simulink model "nl_obsv_hydrotrans_dspace"  (R2021b)
settings: Solver=ode1be  StartTime=0.0  StopTime=inf  FixedStep=ts  MaxStep=ts
PostLoadFcn:
  | if any(exist('dsrtsu_mdlpostloadfcn', 'file') ~= 0), dsrtsu_mdlpostloadfcn('Execute', bdroot); end
InitFcn:
  | , if any(exist('rtifpga_mdlclblib', 'file') ~= 0), rtifpga_mdlclblib('Init', bdroot); end,
  | , if any(exist('dsmpb_private', 'file') ~= 0), dsmpb_private('dsmpb_mdlclblib', 'Init', bdroot); end,
values from neighbouring files (symbols this model uses):
  bd = 5e-2    (= 0.05)    [init_nlobsv_hd.m]
  bf = 0.1    [init_nlobsv_hd.m]
  bm = 0.02    [init_nlobsv_hd.m]
  bp = 0.02    [init_nlobsv_hd.m]
  bulk = 8.36e9    (= 8360000000)    [init_nlobsv_hd.m]
  engine_speed_ref_rpm = 1940    [init_nlobsv_hd.m]
  Jm = 0.05    [init_nlobsv_hd.m]
  Jp = 0.05    [init_nlobsv_hd.m]
  kdrag = 0.01    [init_nlobsv_hd.m]
  kdrag_model = 0.01    [init_nlobsv_hd.m]
  ki_engine = 2.5e-1    (= 0.25)    [init_nlobsv_hd.m]
  kleak = 1e-6    (= 1e-06)    [init_nlobsv_hd.m]
  kp_engine = 2.5e-2    (= 0.025)    [init_nlobsv_hd.m]
  max_domega_m_dt = omega_m_nom_rpm/4    (= 1000)    [init_nlobsv_hd.m]
  ntg = 1    [init_nlobsv_hd.m]
  omega_m_nom_rpm = 4000    [init_nlobsv_hd.m]
  omega_m_ref = 3200    [init_nlobsv_hd.m]
  P0 = eye(4)    [init_nlobsv_hd.m]
  q11 = 10    [init_nlobsv_hd.m]
  q22 = 10    [init_nlobsv_hd.m]
  q33 = 10    [init_nlobsv_hd.m]
  q44 = 2e3    (= 2000)    [init_nlobsv_hd.m]
  ts = 1e-3    (= 0.001)    [init_nlobsv_hd.m]
  tstep = 20    [init_nlobsv_hd.m]
  Vm_nom = 280    [init_nlobsv_hd.m]
  Vp_nom = 210    [init_nlobsv_hd.m]
undefined symbols (not defined in the file or in its folder): consumption, DiscIntNeverNeededParam, rpm_base, rpm_consumption, torque_base, torque_consumption, torque_friction_base
libraries: fl_lib x70, nesl_utility x36, linear_swashplate_ctrl_lib x4, variable_displacement_motor_2_lib x2, variable_displacement_pump_2_lib x2, fixed_displacement_pump_lib x2, relief_valve_lib x2, inverse_shuttle_valve_lib x2, engine_speed_ctrl_kinputs_lib x1, ice_lib x1, gear2_lib x1, flexshaft_lib x1
(part 1 of 2)
PreSaveFcn:
  | , if any(exist('dsmpb_private', 'file') ~= 0), dsmpb_private('dsmpb_mdlclblib', 'PreSave', bdroot); end,
CloseFcn:
  | , if any(exist('dsmpb_private', 'file') ~= 0), dsmpb_private('dsmpb_mdlclblib', 'Close', bdroot); end,
settings Model: RTICANMMDATA=struct('GeneralSetupData',struct('modelroot','C:\Users\dbagn\Dropbox\anno_2022_2023\matlab\anno2022\lectures\nonlinear_obsv_hydrostatic_transmission\2022_08_10','generalsettings',struct('filesettings',struct('destfolder',struct('Name','RTICANMM_FILES','Check',1),'buildfolder',struct('Name','.','Check',1),'AbsDestfolder',struct('Name','C:\Users\dbagn\Dropbox\anno_2022_2023\matlab\anno2022\lectures\nonlinear_obsv_hydrostatic_transmission\2022_08_10\RTICANMM_FILES'),'AbsBuildfolder',struct('Name','C:\Users\dbagn\Dropbox\anno_2022_2023\matlab\anno2022\lectures\nonlinear_obsv_hydrostatic_transmission\2022_08_10'))),'options',struct('addpaths',1,'rmpaths',1,'addtrcexclusion',true,'cannavigator',struct('checkmonitoring',0),'show_usrtrc',0,'use_usrtrc',0),'advanced',struct('options',ones(1,100)),'MPSetup',{{}},'RTI',struct('Type','DSRT','Ver','4.6','Date','02-Nov-2021'),'modelname','nl_obsv_hydrotrans_dspace','block','nl_obsv_hydrotrans_dspace'))  DSRTSU_INTERNAL_RTIFPGA=170  DSRTSU_INTERNAL_RTISTBM_VER=1.4.3  DSMPB_ID_DATA={}  SimulationMode=accelerator  Creator=dbagn  LastModifiedBy=dbagn
settings SolverCC: ZeroCrossAlgorithm=Adaptive
settings DataIOCC: SaveOutput=off  SignalLogging=off  DSMLogging=off  SaveTime=off  ReturnWorkspaceOutputs=off
settings OptimizationCC: BlockReduction=off  ConditionallyExecuteInputs=off  OptimizeBlockIOStorage=off  BufferReuse=off  EnhancedBackFolding=on  PassReuseOutputArgsThreshold=0  OptimizeBlockOrder=speed  DifferentSizesBufferReuse=on
settings DebuggingCC: IgnoredZcDiagnostic=none  TasksWithSamePriorityMsg=none  ParameterTunabilityLossMsg=error
settings HardwareCC: ProdBitPerPointer=32  ProdBitPerSizeT=32  ProdBitPerPtrDiffT=32  ProdLargestAtomicInteger=Integer  ProdWordSize=32  ProdLongLongMode=on  ProdHWDeviceType=Custom Processor->Custom
settings ModelReferenceCC: EnableParallelModelReferenceBuilds=on
settings SFSimCC: MATLABDynamicMemAlloc=off
settings RTWCC: Description=dSPACE Run-Time Target (for VEOS on Windows and ConfigurationDesk)  SystemTargetFile=dsrt.tlc  GenCodeOnly=on  MakeCommand=make_dsrt  TemplateMakefile=dsrt_default_tmf  RTWVerbose=off
settings CodeAppCC: ForceParamTrailComments=on  OperatorAnnotations=on
settings STFCustomTargetCC: TargetLangStandard=C99 (ISO)  ParMdlRefBuildCompliant=on  GRTInterface=off  SystemTargetFile=dsrt.tlc
settings GRTTargetCC: CompOptLevelCompliant=off  ConcurrentExecutionCompliant=off  CombineOutputUpdateFcns=off  MatFileLogging=off  CPPClassGenCompliant=off  UseToolchainInfoCompliant=off

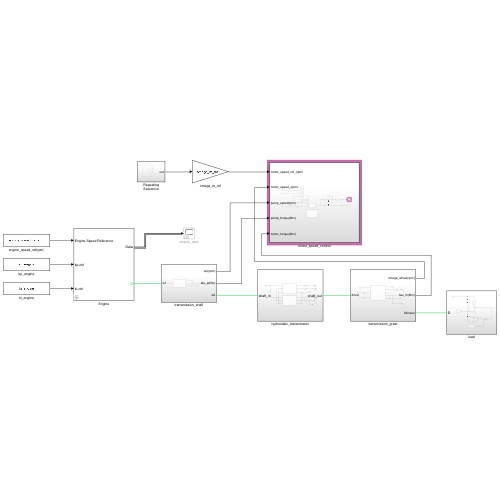
[thumbnail: Simulink's stored preview of the top-level diagram]
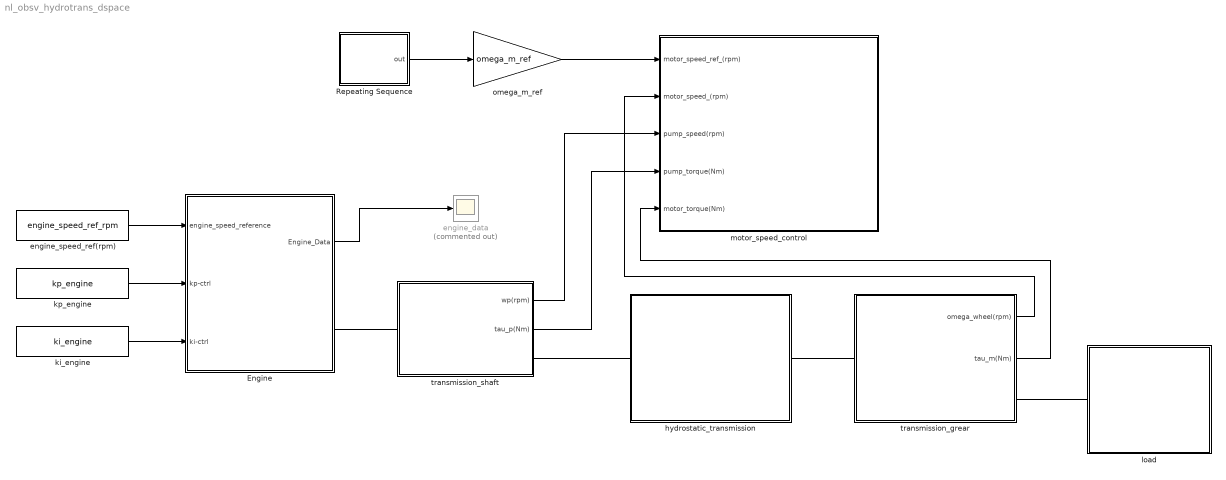
== system nl_obsv_hydrotrans_dspace ==
  Engine : Subsystem  mask(Internal Combustion Engine (ICE)){inertia=7.5, inertia_unit=kg*m^2, init_speed=5, diesel_density=0.85, diesel_density_unit=kg/l, rpm_base=rpm_base, rpm_base_unit=rpm, torque_friction_base=torque_friction_base, torque_friction_base_unit=N*m, torque_base=torque_base, torque_base_unit=N*m, rpm_consumption=rpm_consumption, rpm_consumption_unit=rpm, torque_consumption=torque_consumption, torque_consumption_unit=N*m, consumption=consumption, consumption_unit=g/(kW*hr), kd=0}
      mask prompts: init_speed "Initial Speed (RPM)"; diesel_density "Diesel density"; rpm_base "Base Speed Breakpoints"; torque_friction_base "Base Torque Friction Breakpoints"; torque_base "Base Torque Breakpoints"; rpm_consumption "Speed consumption breakpoints"; torque_consumption "Torque consumption breakpoints"; consumption "Consumption map"
      mask help:
      | This component models a generic internal combustion engine, modelled by means of introducing its characteristic performance maps.
      | Maps of main engine performance and of consumption have to be introduced. The component is also provided with a speed controller in which the PID gains can be introduced.
      mask init:
      | engine = [gcb, '/Generic Internal Combustion Engine'];
      | ctrl = [gcb, '/Engine Speed Controller'];
      | 
      | % Engine Parameters
      | set_param([engine],'cshaft_inertia','inertia');
      | set_param([engine],'cshaft_inertia_unit',inertia_unit);
      | set_param([engine],'initial_speed','init_speed');
      | set_param([engine],'diesel_density','diesel_density');
      | set_param([engine],'diesel_density_unit',diesel_density_unit);
      | 
      | % Tables
      | set_param([engine],'rpm_base','rpm_base');
      | set_param([engine],'torque_friction_base', 'torque_friction_base');
      | set_param([engine],'torque_base','torque_base');
      | set_param([engine],'rpm_consumption','rpm_consumption');
      | set_param([engine],'torque_consumption','torque_consumption');
      | set_param([engine],'consumption','consumption');
      | 
      | set_param([engine],'rpm_base_unit',rpm_base_unit);
      | set_param([engine],'torque_friction_base_unit',torque_friction_base_unit);
      | set_param([engine],'torque_base_unit',torque_base_unit);
      | set_param([engine],'rpm_consumption_unit',rpm_consumption_unit);
      | set_param([engine],'torque_consumption_unit',torque_consumption_unit);
      | set_param([engine],'consumption_unit',consumption_unit);
      | 
      | % Speed control
      | set_param([ctrl],'kd','kd');
      mask Help: eval('open \documentation\liebherr_engine_D9512_model_description.pdf')
      mask TypeOptions inertia_unit: kg*m^2
      mask TypeOptions diesel_density_unit: kg/l
      mask TypeOptions rpm_base_unit: rpm
      mask TypeOptions torque_friction_base_unit: N*m
      mask TypeOptions torque_base_unit: N*m
      mask TypeOptions rpm_consumption_unit: rpm
      mask TypeOptions torque_consumption_unit: kW
      mask TypeOptions consumption_unit: g/(kW*hr)
      mask DialogControl EngineParameters Prompt: Engine Parameters
      mask DialogControl Container5 Prompt: Engine Main Behaviour
      mask DialogControl Container4 Prompt: Consumption Behaviour
      mask DialogControl ControlParameters Prompt: Control Parameters
      mask Display:
      | modelname = [gcb];
      | % image(imread('Complementary/Pics/ICE.jpg'));
      | 
      | % color('red')
      | % port_label('lconn',1,'wref');
      | color('green')
      | port_label('rconn',1,'D');
      | color('black')
      | port_label('output',1,'Data');
      | port_label('input',1,'Engine Speed Reference');
      | port_label('input',2,'kp-ctrl');
      | port_label('input',3,'ki-ctrl');
  Repeating Sequence : Subsystem
  engine_data : Scope  Commented=on
  engine_speed_ref(rpm) : Constant  Value=engine_speed_ref_rpm
  hydrostatic_transmission : Subsystem
  ki_engine : Constant  Value=ki_engine
  kp_engine : Constant  Value=kp_engine
  load : Subsystem
  motor_speed_control : Subsystem
  omega_m_ref : Gain  Gain=omega_m_ref
  transmission_grear : Subsystem
  transmission_shaft : Subsystem
  wires:
  engine_speed_ref(rpm)/1 -> Engine/1(engine_speed_reference)
  Repeating Sequence/1(out) -> omega_m_ref/1
  Engine/1(Engine_Data) -> engine_data/1
  transmission_grear/1(omega_wheel(rpm)) -> motor_speed_control/2(motor_speed_(rpm))
  transmission_shaft/2(tau_p(Nm)) -> motor_speed_control/4(pump_torque(Nm))
  transmission_shaft/1(wp(rpm)) -> motor_speed_control/3(pump_speed(rpm))
  transmission_grear/2(tau_m(Nm)) -> motor_speed_control/5(motor_torque(Nm))
  omega_m_ref/1 -> motor_speed_control/1(motor_speed_ref_(rpm))
  kp_engine/1 -> Engine/2(kp-ctrl)
  ki_engine/1 -> Engine/3(ki-ctrl)
  connections:
  transmission_grear/LConn1 -- hydrostatic_transmission/RConn1
  Engine/RConn1 -- transmission_shaft/LConn1
  transmission_shaft/RConn1 -- hydrostatic_transmission/LConn1
  transmission_grear/RConn1 -- load/LConn1

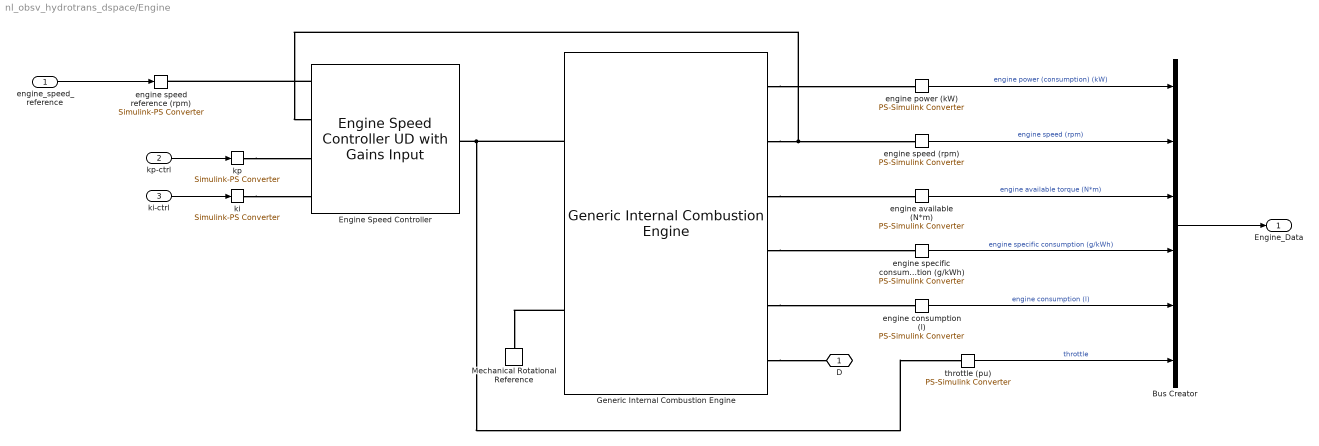
== system nl_obsv_hydrotrans_dspace/Engine ==
  engine_speed_reference : Inport
  kp-ctrl : Inport  Port=2
  ki-ctrl : Inport  Port=3
  Bus Creator : BusCreator  Inputs=6
  Engine Speed Controller : engine_speed_ctrl_kinputs_lib/Engine Speed Controller UD with Gains Input  kd=kd s^2  t_out_specify=off  t_out_priority=None  t_out=0.0  t_out_nominal_specify=off  t_out_nominal_unit=1  t_out_nominal_value=1
      settings: InternalSimscapePortConfiguration="{\"Bottom\":[],\"Left\":[{\"id\":\"we_ref\",\"label\":\"we_ref\",\"type\":\"input\"},{\"id\":\"we\",\"label\":\"we\",\"type\":\"input\"},{\"id\":\"kp\",\"label\":\"kp\",\"type\":\"input\"},{\"id\":\"ki\",\"label\":\"ki\",\"type\":\"input\"}],\"Right\":[{\"id\":\"theta\",\"label\":\"tS\",\"type\":\"output\"}],\"Top\":[]}"
  Generic Internal Combustion Engine : ice_lib/Generic Internal Combustion Engine  cshaft_inertia=inertia kg*m^2  initial_speed=init_speed  diesel_density=diesel_density kg/l  rpm_consumption=rpm_consumption rpm  torque_consumption=torque_consumption N*m  consumption=consumption g/(kW*hr)  rpm_base=rpm_base rpm  torque_friction_base=torque_friction_base N*m  torque_base=torque_base N*m
      settings: InternalSimscapePortConfiguration="{\"Bottom\":[],\"Left\":[{\"id\":\"theta\",\"label\":\"theta\",\"type\":\"input\"},{\"id\":\"C\",\"label\":\"C\",\"type\":\"foundation.mechanical.rotational.rotational\"}],\"Right\":[{\"id\":\"Pe\",\"label\":\"Pe\",\"type\":\"output\"},{\"id\":\"omega_e_out\",\"label\":\"omega_e\",\"type\":\"output\"},{\"id\":\"tau_d_out\",\"label\":\"tau_d\",\"type\":\"output\"},{\"id\":\"sfc\",\"label\":\"sfc\",\"type\":\"output\"},{\"id\":\"fc\",\"label\":\"fc\",\"type\":\"output\"},{\"id\":\"D\",\"label\":\"D\",\"type\":\"foundation.mechanical.rotational.rotational\"}],\"Top\":[]}"
  Mechanical Rotational Reference : fl_lib/Mechanical/Rotational Elements/Mechanical Rotational Reference
  engine available (N*m) : nesl_utility/PS-Simulink Converter  PhysicalDomain=network_engine_domain  SubClassName=ps_output  LeftPortType=input  RightPortType=output  PseudoPeriodic=off  Frequencies=[]  Unit=N*m  AffineConversion=on
      settings: SourceProductBaseCode=PW,SS
  engine consumption (l) : nesl_utility/PS-Simulink Converter  PhysicalDomain=network_engine_domain  SubClassName=ps_output  LeftPortType=input  RightPortType=output  PseudoPeriodic=off  Frequencies=[]  Unit=l  AffineConversion=on
      settings: SourceProductBaseCode=PW,SS
  engine power (kW) : nesl_utility/PS-Simulink Converter  PhysicalDomain=network_engine_domain  SubClassName=ps_output  LeftPortType=input  RightPortType=output  PseudoPeriodic=off  Frequencies=[]  Unit=kW  AffineConversion=on
      settings: SourceProductBaseCode=PW,SS
  engine specific consumption (g/kWh) : nesl_utility/PS-Simulink Converter  PhysicalDomain=network_engine_domain  SubClassName=ps_output  LeftPortType=input  RightPortType=output  PseudoPeriodic=off  Frequencies=[]  Unit=g/(kW*hr)  AffineConversion=on
      settings: SourceProductBaseCode=PW,SS
  engine speed (rpm) : nesl_utility/PS-Simulink Converter  PhysicalDomain=network_engine_domain  SubClassName=ps_output  LeftPortType=input  RightPortType=output  PseudoPeriodic=off  Frequencies=[]  Unit=rpm  AffineConversion=on
      settings: SourceProductBaseCode=PW,SS
  engine speed reference (rpm) : nesl_utility/Simulink-PS Converter  PhysicalDomain=network_engine_domain  SubClassName=ps_input  LeftPortType=input  RightPortType=output  PseudoPeriodic=off  Frequencies=[]  NoiseDistribution=none  NoiseParameters=[]  Unit=rpm  AffineConversion=on  FilteringAndDerivatives=provide  SimscapeFilterOrder=1  InputFilterTimeConstant=0.001  UdotUserProvided=0
      settings: SourceProductBaseCode=PW,SS
  ki : nesl_utility/Simulink-PS Converter  PhysicalDomain=network_engine_domain  SubClassName=ps_input  LeftPortType=input  RightPortType=output  PseudoPeriodic=off  Frequencies=[]  NoiseDistribution=none  NoiseParameters=[]  Unit=1  AffineConversion=on  FilteringAndDerivatives=provide  SimscapeFilterOrder=1  InputFilterTimeConstant=0.001  UdotUserProvided=0
      settings: SourceProductBaseCode=PW,SS
  kp : nesl_utility/Simulink-PS Converter  PhysicalDomain=network_engine_domain  SubClassName=ps_input  LeftPortType=input  RightPortType=output  PseudoPeriodic=off  Frequencies=[]  NoiseDistribution=none  NoiseParameters=[]  Unit=s  AffineConversion=on  FilteringAndDerivatives=provide  SimscapeFilterOrder=1  InputFilterTimeConstant=0.001  UdotUserProvided=0
      settings: SourceProductBaseCode=PW,SS
  throttle (pu) : nesl_utility/PS-Simulink Converter  PhysicalDomain=network_engine_domain  SubClassName=ps_output  LeftPortType=input  RightPortType=output  PseudoPeriodic=off  Frequencies=[]  Unit=1  AffineConversion=on
      settings: SourceProductBaseCode=PW,SS
  D : PMIOPort  Side=Right
  Engine_Data : Outport
  wires:
  engine speed (rpm)/1 -> Bus Creator/2  "engine speed (rpm)"
  engine specific consumption (g/kWh)/1 -> Bus Creator/4  "engine specific consumption (g/kWh)"
  engine available (N*m)/1 -> Bus Creator/3  "engine available torque (N*m)"
  Bus Creator/1 -> Engine_Data/1
  engine consumption (l)/1 -> Bus Creator/5  "engine consumption (l)"
  engine power (kW)/1 -> Bus Creator/1  "engine power (consumption) (kW)"
  throttle (pu)/1 -> Bus Creator/6  "throttle"
  engine_speed_reference/1 -> engine speed reference (rpm)/1
  kp-ctrl/1 -> kp/1
  ki-ctrl/1 -> ki/1
  connections:
  Generic Internal Combustion Engine/LConn2 -- Mechanical Rotational Reference/LConn1
  Generic Internal Combustion Engine/RConn1 -- engine power (kW)/LConn1
  Generic Internal Combustion Engine/RConn6 -- D/RConn1
  Generic Internal Combustion Engine/RConn2 -- Engine Speed Controller/LConn2 -- engine speed (rpm)/LConn1
  Generic Internal Combustion Engine/RConn4 -- engine specific consumption (g/kWh)/LConn1
  Generic Internal Combustion Engine/RConn3 -- engine available (N*m)/LConn1
  Generic Internal Combustion Engine/LConn1 -- throttle (pu)/LConn1 -- Engine Speed Controller/RConn1
  Generic Internal Combustion Engine/RConn5 -- engine consumption (l)/LConn1
  Engine Speed Controller/LConn1 -- engine speed reference (rpm)/RConn1
  kp/RConn1 -- Engine Speed Controller/LConn3
  ki/RConn1 -- Engine Speed Controller/LConn4

== system nl_obsv_hydrotrans_dspace/Repeating Sequence ==
  Constant : Constant  Value=-1
  Constant1 : Constant
  Constant2 : Constant  Value=0
  Constant3 : Constant
  Constant4 : Constant
  Discrete-Time Integrator : DiscreteIntegrator  IntegratorMethod=Integration: Backward Euler  ExternalReset=rising  SampleTime=-1  ICPrevOutput=DiscIntNeverNeededParam  ICPrevScaledInput=DiscIntNeverNeededParam
  Switch : Switch  Criteria=u2 > Threshold  Threshold=tstep
  Switch1 : Switch  Criteria=u2 > Threshold  Threshold=2*tstep
  Unit Delay : UnitDelay  SampleTime=ts  HasFrameUpgradeWarning=on
  out : Outport
  wires:
  Constant4/1 -> Discrete-Time Integrator/1
  Constant/1 -> Switch/1
  Discrete-Time Integrator/1 -> Switch1/2, Switch/2
  Constant3/1 -> Switch1/1
  Constant1/1 -> Switch/3
  Constant2/1 -> Switch1/3
  Switch1/1 -> Unit Delay/1
  Unit Delay/1 -> Discrete-Time Integrator/2
  Switch/1 -> out/1

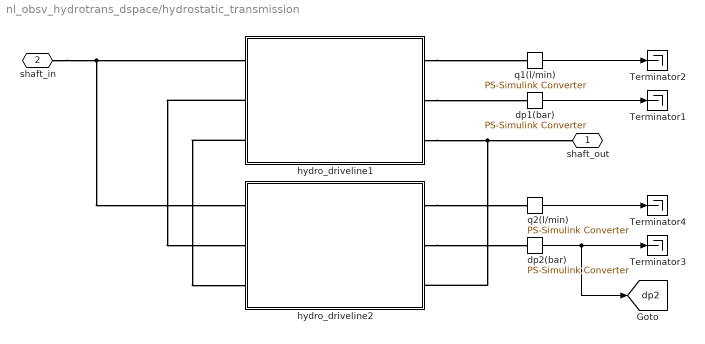
== system nl_obsv_hydrotrans_dspace/hydrostatic_transmission ==
  Terminator{1..4} (4 alike) : Terminator
  dp1(bar) : nesl_utility/PS-Simulink Converter  PhysicalDomain=network_engine_domain  SubClassName=ps_output  LeftPortType=input  RightPortType=output  PseudoPeriodic=off  Frequencies=[]  Unit=bar  AffineConversion=off
      settings: SourceProductBaseCode=PW,SS
  dp2(bar) : nesl_utility/PS-Simulink Converter  PhysicalDomain=network_engine_domain  SubClassName=ps_output  LeftPortType=input  RightPortType=output  PseudoPeriodic=off  Frequencies=[]  Unit=bar  AffineConversion=off
      settings: SourceProductBaseCode=PW,SS
  hydro_driveline1 : Subsystem
  hydro_driveline2 : Subsystem
  q1(l/min) : nesl_utility/PS-Simulink Converter  PhysicalDomain=network_engine_domain  SubClassName=ps_output  LeftPortType=input  RightPortType=output  PseudoPeriodic=off  Frequencies=[]  Unit=l/min  AffineConversion=on
      settings: SourceProductBaseCode=PW,SS
  q2(l/min) : nesl_utility/PS-Simulink Converter  PhysicalDomain=network_engine_domain  SubClassName=ps_output  LeftPortType=input  RightPortType=output  PseudoPeriodic=off  Frequencies=[]  Unit=l/min  AffineConversion=on
      settings: SourceProductBaseCode=PW,SS
  shaft_out : PMIOPort  Side=Right
  shaft_in : PMIOPort  Port=2  Side=Left
  tag scope: dp2=global
  wires:
  q1(l/min)/1 -> Terminator2/1
  dp1(bar)/1 -> Terminator1/1
  dp2(bar)/1 -> Terminator3/1, [dp2]
  q2(l/min)/1 -> Terminator4/1
  connections:
  shaft_in/RConn1 -- hydro_driveline1/LConn1 -- hydro_driveline2/LConn1
  hydro_driveline1/RConn1 -- q1(l/min)/LConn1
  hydro_driveline1/RConn2 -- dp1(bar)/LConn1
  hydro_driveline1/RConn3 -- hydro_driveline2/RConn3 -- shaft_out/RConn1
  hydro_driveline1/LConn2 -- hydro_driveline2/LConn2
  hydro_driveline1/LConn3 -- hydro_driveline2/LConn3
  hydro_driveline2/RConn1 -- q2(l/min)/LConn1
  hydro_driveline2/RConn2 -- dp2(bar)/LConn1

== system nl_obsv_hydrotrans_dspace/load ==
  Ideal Rotational Motion Sensor : fl_lib/Mechanical/Mechanical Sensors/Ideal Rotational Motion Sensor  wrap_angle=simscape.enum.onoff.off  offset=0 rad
  Ideal Torque Source : fl_lib/Mechanical/Mechanical Sources/Ideal Torque Source
  Mechanical Rotational Reference : fl_lib/Mechanical/Rotational Elements/Mechanical Rotational Reference
  PS Product : fl_lib/Physical Signals/Functions/PS Product
  PS Product1 : fl_lib/Physical Signals/Functions/PS Product
  PS Product2 : fl_lib/Physical Signals/Functions/PS Product
  PS Sign : fl_lib/Physical Signals/Nonlinear Operators/PS Sign
      settings: SourceProductBaseCode=SS  InternalSimscapePortConfiguration="{\"Bottom\":[],\"Left\":[{\"id\":\"I\",\"label\":\"\",\"type\":\"input\"}],\"Right\":[{\"id\":\"O\",\"label\":\"\",\"type\":\"output\"}],\"Top\":[]}"
  Solver Configuration : nesl_utility/Solver Configuration  PhysicalDomain=network_engine_domain  SubClassName=solver  LeftPortType=input  RightPortType=generic  Tones=[]  Harmonics=[]  SimulateNoise=off  Profile=off  UseLocalSampling=off  EnableSwitchedLinearOptims=on  FrequencyDomain=off  UseCCode=off  RelTol=0.001  AbsTol=1e-06  MinStep=1e-09  ToWorkspace=off  RevertToSquareIcSolve=off  NumHomotopyIterations=100  PhasorMode=off  PhasorModeNumHarmonics=1  DoDC=off  ResidualTolerance=ts  UseLocalSolver=on  LocalSolverChoice=NE_BACKWARD_EULER_ADVANCER  LocalSolverSampleTime=ts  DoFixedCost=on  MaxNonlinIter=3  MaxModeIter=2  ComputeImpulses=off  ImpulseIterations=2  LinearAlgebra=auto  EquationFormulation=NE_TIME_EF  DelaysMemoryBudget=1024  AutomaticFiltering=on  FilteringTimeConstant=ts  PartitionStorageMethod=AS_NEEDED  PartitionMemoryBudget=1024  PartitionMethod=ROBUST
      settings: SourceProductBaseCode=PW,SS
  kdrag : Constant  Value=-kdrag
  kdrag_converter : nesl_utility/Simulink-PS Converter  PhysicalDomain=network_engine_domain  SubClassName=ps_input  LeftPortType=input  RightPortType=output  PseudoPeriodic=off  Frequencies=[]  NoiseDistribution=none  NoiseParameters=[]  Unit=N*m/(rad/s)^2  AffineConversion=on  FilteringAndDerivatives=provide  SimscapeFilterOrder=1  InputFilterTimeConstant=0.001  UdotUserProvided=0
      settings: SourceProductBaseCode=PW,SS
  D : PMIOPort  Side=Left
  wires:
  kdrag/1 -> kdrag_converter/1
  connections:
  PS Product1/LConn1 -- PS Product/RConn1
  Ideal Rotational Motion Sensor/RConn1 -- Solver Configuration/RConn1 -- Mechanical Rotational Reference/LConn1 -- Ideal Torque Source/RConn2
  PS Sign/RConn1 -- PS Product1/LConn2
  Ideal Torque Source/LConn1 -- D/RConn1 -- Ideal Rotational Motion Sensor/LConn1
  Ideal Torque Source/RConn1 -- PS Product2/RConn1
  Ideal Rotational Motion Sensor/RConn2 -- PS Product/LConn2 -- PS Product/LConn1 -- PS Sign/LConn1
  PS Product2/LConn1 -- PS Product1/RConn1
  kdrag_converter/RConn1 -- PS Product2/LConn2

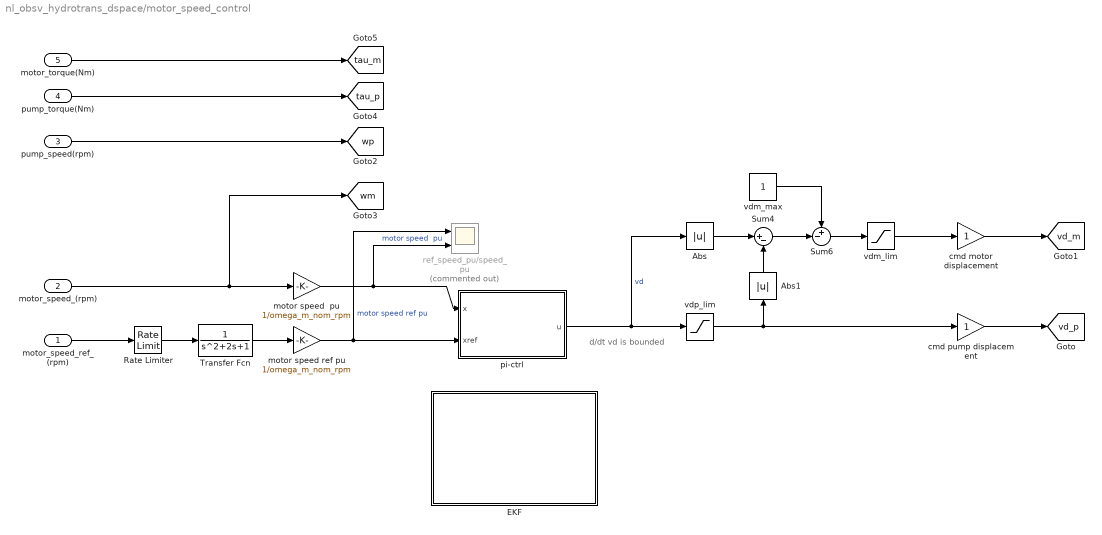
== system nl_obsv_hydrotrans_dspace/motor_speed_control ==
  note: d/dt vd is bounded
  motor_speed_ref_(rpm) : Inport
  motor_speed_(rpm) : Inport  Port=2
  pump_speed(rpm) : Inport  Port=3
  pump_torque(Nm) : Inport  Port=4
  motor_torque(Nm) : Inport  Port=5
  Abs : Abs
  Abs1 : Abs
  EKF : Subsystem
  Rate Limiter : RateLimiter  RisingSlewLimit=max_domega_m_dt  FallingSlewLimit=-max_domega_m_dt  SampleTimeMode=inherited
  Sum4 : Sum  Inputs=|+-
  Sum6 : Sum  Inputs=+-|
  Transfer Fcn : TransferFcn
  cmd motor displacement : Gain
  cmd pump displacement : Gain
  motor speed  pu : Gain  Gain=1/omega_m_nom_rpm
  motor speed ref pu : Gain  Gain=1/omega_m_nom_rpm
  pi-ctrl : Subsystem  mask{kp=1, ki=18, ts=ts, sat_pos=1.64, sat_neg=-1.64}
  ref_speed_pu/speed_pu : Scope  Commented=on  NumInputPorts=2
  vdm_lim : Saturate  UpperLimit=1  LowerLimit=0.36
  vdm_max : Constant
  vdp_lim : Saturate  UpperLimit=1  LowerLimit=-1
  tag scope: tau_m=global, tau_p=global, vd_m=global, vd_p=global, wm=global, wp=global
  wires:
  motor speed ref pu/1 -> ref_speed_pu/speed_pu/1, pi-ctrl/2(xref)  "motor speed ref pu"
  vdp_lim/1 -> cmd pump displacement/1, Abs1/1
  vdm_lim/1 -> cmd motor displacement/1
  Sum4/1 -> Sum6/2
  motor_speed_(rpm)/1 -> [wm], motor speed  pu/1
  motor_speed_ref_(rpm)/1 -> Rate Limiter/1
  Abs1/1 -> Sum4/2
  Sum6/1 -> vdm_lim/1
  vdm_max/1 -> Sum6/1
  Abs/1 -> Sum4/1
  motor speed  pu/1 -> ref_speed_pu/speed_pu/2, pi-ctrl/1(x)  "motor speed  pu"
  Transfer Fcn/1 -> motor speed ref pu/1
  pi-ctrl/1(u) -> Abs/1, vdp_lim/1  "vd"
  pump_speed(rpm)/1 -> [wp]
  Rate Limiter/1 -> Transfer Fcn/1
  pump_torque(Nm)/1 -> [tau_p]
  motor_torque(Nm)/1 -> [tau_m]
  cmd motor displacement/1 -> [vd_m]
  cmd pump displacement/1 -> [vd_p]

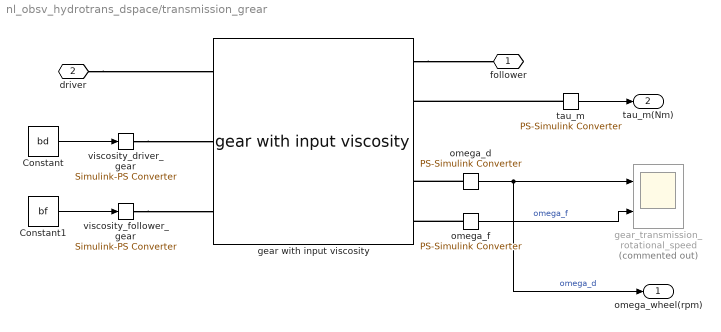
== system nl_obsv_hydrotrans_dspace/transmission_grear ==
  Constant : Constant  Value=bd
  Constant1 : Constant  Value=bf
  gear with input viscosity : gear2_lib/gear with input viscosity  n1=1  n2=1  J1=Jd kg*m^2  J2=Jf kg*m^2  k_theta_1=k_theta_tg N*m/rad  w_1_specify=off  w_1_priority=None  w_1=0 rad/s  w_1_nominal_specify=off  w_1_nominal_unit=rad/s  w_1_nominal_value=1  w_2_specify=off  w_2_priority=None  w_2=0 rad/s  w_2_nominal_specify=off  w_2_nominal_unit=rad/s  w_2_nominal_value=1  t_1_specify=off  t_1_priority=None  t_1=0 N*m  t_1_nominal_specify=off  t_1_nominal_unit=N*m  t_1_nominal_value=1  t_2_specify=off  t_2_priority=None  t_2=0 N*m  t_2_nominal_specify=off  t_2_nominal_unit=N*m  t_2_nominal_value=1  t_theta_1_specify=off  t_theta_1_priority=None  t_theta_1=0 N*m  t_theta_1_nominal_specify=off  t_theta_1_nominal_unit=N*m  t_theta_1_nominal_value=1  t_theta_2_specify=off  t_theta_2_priority=None  t_theta_2=0 N*m  t_theta_2_nominal_specify=off  t_theta_2_nominal_unit=N*m  t_theta_2_nominal_value=1
      settings: InternalSimscapePortConfiguration="{\"Bottom\":[],\"Left\":[{\"id\":\"S1\",\"label\":\"S1\",\"type\":\"foundation.mechanical.rotational.rotational\"},{\"id\":\"b1\",\"label\":\"b1\",\"type\":\"input\"},{\"id\":\"b2\",\"label\":\"b2\",\"type\":\"input\"}],\"Right\":[{\"id\":\"S2\",\"label\":\"S2\",\"type\":\"foundation.mechanical.rotational.rotational\"},{\"id\":\"tau_theta_1\",\"label\":\"tau_theta_1\",\"type\":\"output\"},{\"id\":\"tau_theta_2\",\"label\":\"tau_theta_2\",\"type\":\"output\"},{\"id\":\"w1\",\"label\":\"w1\",\"type\":\"output\"},{\"id\":\"w2\",\"label\":\"w2\",\"type\":\"output\"}],\"Top\":[]}"
  gear_transmission_rotational_speed : Scope  Commented=on  NumInputPorts=2
  omega_d : nesl_utility/PS-Simulink Converter  PhysicalDomain=network_engine_domain  SubClassName=ps_output  LeftPortType=input  RightPortType=output  PseudoPeriodic=off  Frequencies=[]  Unit=rpm  AffineConversion=on
      settings: SourceProductBaseCode=PW,SS
  omega_f : nesl_utility/PS-Simulink Converter  PhysicalDomain=network_engine_domain  SubClassName=ps_output  LeftPortType=input  RightPortType=output  PseudoPeriodic=off  Frequencies=[]  Unit=rpm  AffineConversion=on
      settings: SourceProductBaseCode=PW,SS
  tau_m : nesl_utility/PS-Simulink Converter  PhysicalDomain=network_engine_domain  SubClassName=ps_output  LeftPortType=input  RightPortType=output  PseudoPeriodic=off  Frequencies=[]  Unit=N*m  AffineConversion=on
      settings: SourceProductBaseCode=PW,SS
  viscosity_driver_gear : nesl_utility/Simulink-PS Converter  PhysicalDomain=network_engine_domain  SubClassName=ps_input  LeftPortType=input  RightPortType=output  PseudoPeriodic=off  Frequencies=[]  NoiseDistribution=none  NoiseParameters=[]  Unit=(N*m)*(s/rad)  AffineConversion=on  FilteringAndDerivatives=provide  SimscapeFilterOrder=1  InputFilterTimeConstant=0.001  UdotUserProvided=0
      settings: SourceProductBaseCode=PW,SS
  viscosity_follower_gear : nesl_utility/Simulink-PS Converter  PhysicalDomain=network_engine_domain  SubClassName=ps_input  LeftPortType=input  RightPortType=output  PseudoPeriodic=off  Frequencies=[]  NoiseDistribution=none  NoiseParameters=[]  Unit=(N*m)*(s/rad)  AffineConversion=on  FilteringAndDerivatives=provide  SimscapeFilterOrder=1  InputFilterTimeConstant=0.001  UdotUserProvided=0
      settings: SourceProductBaseCode=PW,SS
  follower : PMIOPort  Side=Right
  driver : PMIOPort  Port=2  Side=Left
  omega_wheel(rpm) : Outport
  tau_m(Nm) : Outport  Port=2
  wires:
  Constant/1 -> viscosity_driver_gear/1
  Constant1/1 -> viscosity_follower_gear/1
  omega_d/1 -> omega_wheel(rpm)/1, gear_transmission_rotational_speed/1  "omega_d"
  omega_f/1 -> gear_transmission_rotational_speed/2  "omega_f"
  tau_m/1 -> tau_m(Nm)/1
  connections:
  viscosity_follower_gear/RConn1 -- gear with input viscosity/LConn3
  viscosity_driver_gear/RConn1 -- gear with input viscosity/LConn2
  gear with input viscosity/RConn1 -- follower/RConn1
  omega_d/LConn1 -- gear with input viscosity/RConn4
  omega_f/LConn1 -- gear with input viscosity/RConn5
  tau_m/LConn1 -- gear with input viscosity/RConn2
  driver/RConn1 -- gear with input viscosity/LConn1

== system nl_obsv_hydrotrans_dspace/transmission_shaft ==
  dir : Gain  Gain=-1
  flexible shaft : flexshaft_lib/flexible shaft  b1=b1 N*m/(rad/s)  J1=J1 kg*m^2  b2=b2 N*m/(rad/s)  J2=J2 kg*m^2  b_theta=b_theta N*m/(rad/s)  k_theta=k_theta N*m/rad  w_1_specify=off  w_1_priority=None  w_1=0 rad/s  w_1_nominal_specify=off  w_1_nominal_unit=rad/s  w_1_nominal_value=1  w_2_specify=off  w_2_priority=None  w_2=0 rad/s  w_2_nominal_specify=off  w_2_nominal_unit=rad/s  w_2_nominal_value=1  t_1_specify=off  t_1_priority=None  t_1=0 N*m  t_1_nominal_specify=off  t_1_nominal_unit=N*m  t_1_nominal_value=1  t_2_specify=off  t_2_priority=None  t_2=0 N*m  t_2_nominal_specify=off  t_2_nominal_unit=N*m  t_2_nominal_value=1  t_theta_specify=off  t_theta_priority=None  t_theta=0 N*m  t_theta_nominal_specify=off  t_theta_nominal_unit=N*m  t_theta_nominal_value=1
      settings: InternalSimscapePortConfiguration="{\"Bottom\":[],\"Left\":[{\"id\":\"S1\",\"label\":\"S1\",\"type\":\"foundation.mechanical.rotational.rotational\"}],\"Right\":[{\"id\":\"S2\",\"label\":\"S2\",\"type\":\"foundation.mechanical.rotational.rotational\"},{\"id\":\"tau2\",\"label\":\"tau2\",\"type\":\"output\"},{\"id\":\"w2\",\"label\":\"w2\",\"type\":\"output\"}],\"Top\":[]}"
  load_speed(rpm) : nesl_utility/PS-Simulink Converter  PhysicalDomain=network_engine_domain  SubClassName=ps_output  LeftPortType=input  RightPortType=output  PseudoPeriodic=off  Frequencies=[]  Unit=rpm  AffineConversion=on
      settings: SourceProductBaseCode=PW,SS
  load_torque(Nm) : nesl_utility/PS-Simulink Converter  PhysicalDomain=network_engine_domain  SubClassName=ps_output  LeftPortType=input  RightPortType=output  PseudoPeriodic=off  Frequencies=[]  Unit=N*m  AffineConversion=on
      settings: SourceProductBaseCode=PW,SS
  w1 : PMIOPort  Side=Left
  w2 : PMIOPort  Port=2  Side=Right
  wp(rpm) : Outport
  tau_p(Nm) : Outport  Port=2
  wires:
  load_speed(rpm)/1 -> wp(rpm)/1
  load_torque(Nm)/1 -> dir/1
  dir/1 -> tau_p(Nm)/1
  connections:
  flexible shaft/RConn1 -- w2/RConn1
  w1/RConn1 -- flexible shaft/LConn1
  load_torque(Nm)/LConn1 -- flexible shaft/RConn2
  load_speed(rpm)/LConn1 -- flexible shaft/RConn3

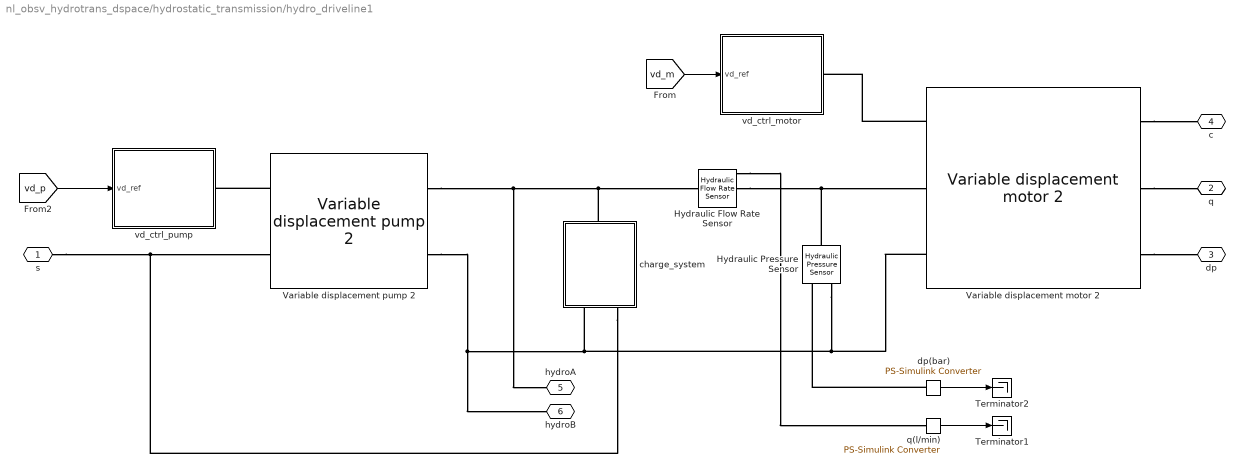
== system nl_obsv_hydrotrans_dspace/hydrostatic_transmission/hydro_driveline1 ==
  Hydraulic Flow Rate Sensor : fl_lib/Hydraulic/Hydraulic Sensors/Hydraulic Flow Rate Sensor
  Hydraulic Pressure Sensor : fl_lib/Hydraulic/Hydraulic Sensors/Hydraulic Pressure Sensor
  Terminator1 : Terminator
  Terminator2 : Terminator
  Variable displacement motor 2 : variable_displacement_motor_2_lib/Variable displacement motor 2  max_Dv=Vm_nom cm^3/rev  min_Dv=20 cm^3/rev  inertia_motor=Jm kg*m^2  oil_vol=4.1 l  bulk=bulk Pa  bp=bm N*m*s/rad  lk=1e-6 m  t_specify=off  t_priority=None  t=0 N*m  t_nominal_specify=off  t_nominal_unit=N*m  t_nominal_value=1  q_specify=off  q_priority=None  q=0 m^3/s  q_nominal_specify=off  q_nominal_unit=m^3/s  q_nominal_value=1  qt_specify=off  qt_priority=None  qt=0 m^3/s  qt_nominal_specify=off  qt_nominal_unit=m^3/s  qt_nominal_value=1  qleak_specify=off  qleak_priority=None  qleak=0 m^3/s  qleak_nominal_specify=off  qleak_nominal_unit=m^3/s  qleak_nominal_value=1  Dv_specify=off  Dv_priority=None  Dv=0 cm^3/rev  Dv_nominal_specify=off  Dv_nominal_unit=cm^3/rev  Dv_nominal_value=1  dp_specify=off  dp_priority=None  dp=0 Pa  dp_nominal_specify=off  dp_nominal_unit=Pa  dp_nominal_value=1  wm_specify=off  wm_priority=None  wm=0 rad/s  wm_nominal_specify=off  wm_nominal_unit=rad/s  wm_nominal_value=1
      settings: InternalSimscapePortConfiguration="{\"Bottom\":[],\"Left\":[{\"id\":\"Vd\",\"label\":\"Vd\",\"type\":\"input\"},{\"id\":\"A\",\"label\":\"A\",\"type\":\"foundation.hydraulic.hydraulic\"},{\"id\":\"B\",\"label\":\"B\",\"type\":\"foundation.hydraulic.hydraulic\"}],\"Right\":[{\"id\":\"C\",\"label\":\"C\",\"type\":\"foundation.mechanical.rotational.rotational\"},{\"id\":\"q_out\",\"label\":\"q\",\"type\":\"output\"},{\"id\":\"delta_p_out\",\"label\":\"dp\",\"type\":\"output\"}],\"Top\":[]}"
  Variable displacement pump 2 : variable_displacement_pump_2_lib/Variable displacement pump 2  max_Dv=Vp_nom cm^3/rev  inertia_pump=Jp kg*m^2  oil_vol=3.0 l  bulk=bulk Pa  bp=bp N*m*s/rad  lk=1e-6 m  t_specify=off  t_priority=None  t=0 N*m  t_nominal_specify=off  t_nominal_unit=N*m  t_nominal_value=1  q_specify=off  q_priority=None  q=0 m^3/s  q_nominal_specify=off  q_nominal_unit=m^3/s  q_nominal_value=1  qt_specify=off  qt_priority=None  qt=0 m^3/s  qt_nominal_specify=off  qt_nominal_unit=m^3/s  qt_nominal_value=1  qleak_specify=off  qleak_priority=None  qleak=0 m^3/s  qleak_nominal_specify=off  qleak_nominal_unit=m^3/s  qleak_nominal_value=1  Dv_specify=off  Dv_priority=None  Dv=0 cm^3/rev  Dv_nominal_specify=off  Dv_nominal_unit=cm^3/rev  Dv_nominal_value=1  dp_specify=off  dp_priority=None  dp=0 Pa  dp_nominal_specify=off  dp_nominal_unit=Pa  dp_nominal_value=1  we_specify=off  we_priority=None  we=0 rad/s  we_nominal_specify=off  we_nominal_unit=rad/s  we_nominal_value=1
      settings: InternalSimscapePortConfiguration="{\"Bottom\":[],\"Left\":[{\"id\":\"Vd\",\"label\":\"Vd\",\"type\":\"input\"},{\"id\":\"C\",\"label\":\"C\",\"type\":\"foundation.mechanical.rotational.rotational\"}],\"Right\":[{\"id\":\"A\",\"label\":\"A\",\"type\":\"foundation.hydraulic.hydraulic\"},{\"id\":\"B\",\"label\":\"B\",\"type\":\"foundation.hydraulic.hydraulic\"}],\"Top\":[]}"
  charge_system : Subsystem
      settings: PortSchema="{\"entries\":[{\"content\":{\"sides\":[{\"content\":{\"connectorIds\":[]},\"type\":\"ConnectorPlacement.EquallySpacedRectSide\",\"uuid\":\"e48dc60c-7abd-410a-894b-273047c8aadd\"},{\"content\":{\"connectorIds\":[],\"side\":\"RIGHT\"},\"type\":\"ConnectorPlacement.EquallySpacedRectSide\",\"uuid\":\"1866d745-b28e-4187-be81-03bff766c239\"},{\"content\":{\"connectorIds\":[\"LConn1\"],\"side\":\"TOP\"},\"type\":\"ConnectorPlacement.EquallySpacedRectSide\",\"uuid\":\"a7856f22-1a7f-4c46-a37a-59c4b01a6b79\"},{\"content\":{\"connectorIds\":[\"RConn1\",\"RConn2\"],\"side\":\"BOTTOM\"},\"type\":\"ConnectorPlacement.EquallySpacedRectSide\",\"uuid\":\"6254cc6e-0892-4919-86d5-0180151530d1\"}]},\"type\":\"ConnectorPlacement.EquallySpacedConnector\",\"uuid\":\"a983534e-afc0-4bb2-9b1c-06b03353b26b\"}],\"packageUris\":[\"http://schema.mathworks.com/mf0/Connector/19700101\"],\"version\":\"1.0\"}"
  dp(bar) : nesl_utility/PS-Simulink Converter  PhysicalDomain=network_engine_domain  SubClassName=ps_output  LeftPortType=input  RightPortType=output  PseudoPeriodic=off  Frequencies=[]  Unit=bar  AffineConversion=on
      settings: SourceProductBaseCode=PW,SS
  q(l/min) : nesl_utility/PS-Simulink Converter  PhysicalDomain=network_engine_domain  SubClassName=ps_output  LeftPortType=input  RightPortType=output  PseudoPeriodic=off  Frequencies=[]  Unit=l/min  AffineConversion=on
      settings: SourceProductBaseCode=PW,SS
  vd_ctrl_motor : Subsystem
  vd_ctrl_pump : Subsystem
  s : PMIOPort  Side=Left
  q : PMIOPort  Port=2  Side=Right
  dp : PMIOPort  Port=3  Side=Right
  c : PMIOPort  Port=4  Side=Right
  hydroA : PMIOPort  Port=5  Side=Left
  hydroB : PMIOPort  Port=6  Side=Left
  wires:
  [vd_m] -> vd_ctrl_motor/1(vd_ref)
  [vd_p] -> vd_ctrl_pump/1(vd_ref)
  dp(bar)/1 -> Terminator2/1
  q(l/min)/1 -> Terminator1/1
  connections:
  Variable displacement motor 2/LConn3 -- Hydraulic Pressure Sensor/RConn1 -- Variable displacement pump 2/RConn2 -- hydroB/RConn1 -- charge_system/RConn1
  s/RConn1 -- Variable displacement pump 2/LConn2 -- charge_system/RConn2
  Variable displacement motor 2/LConn1 -- vd_ctrl_motor/RConn1
  Hydraulic Pressure Sensor/LConn1 -- Hydraulic Flow Rate Sensor/RConn2 -- Variable displacement motor 2/LConn2
  Variable displacement pump 2/LConn1 -- vd_ctrl_pump/RConn1
  Variable displacement motor 2/RConn2 -- q/RConn1
  Variable displacement motor 2/RConn1 -- c/RConn1
  Variable displacement motor 2/RConn3 -- dp/RConn1
  dp(bar)/LConn1 -- Hydraulic Pressure Sensor/RConn2
  Variable displacement pump 2/RConn1 -- hydroA/RConn1 -- charge_system/LConn1 -- Hydraulic Flow Rate Sensor/LConn1
  Hydraulic Flow Rate Sensor/RConn1 -- q(l/min)/LConn1

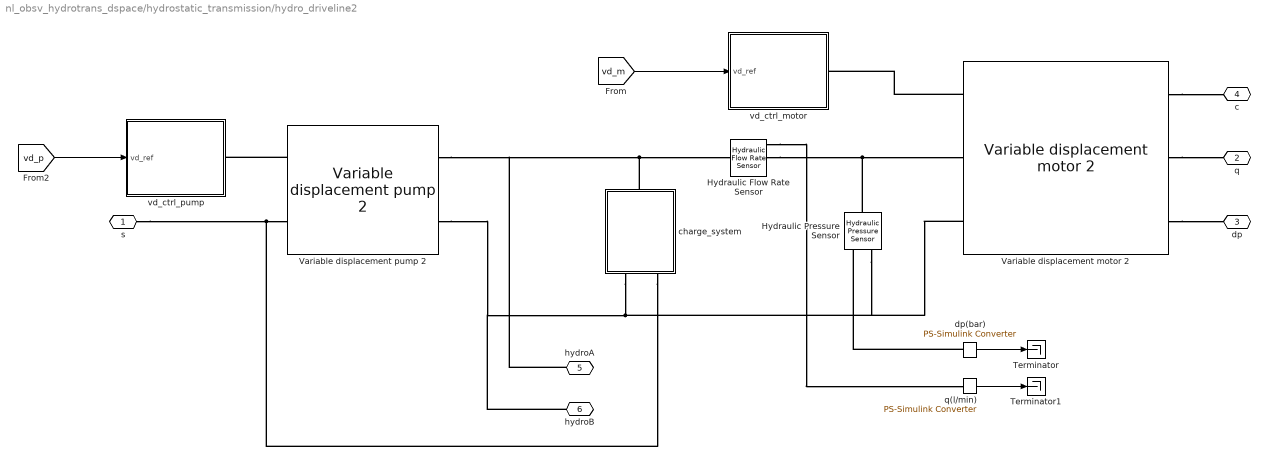
== system nl_obsv_hydrotrans_dspace/hydrostatic_transmission/hydro_driveline2 ==
  Hydraulic Flow Rate Sensor : fl_lib/Hydraulic/Hydraulic Sensors/Hydraulic Flow Rate Sensor
  Hydraulic Pressure Sensor : fl_lib/Hydraulic/Hydraulic Sensors/Hydraulic Pressure Sensor
  Terminator : Terminator
  Terminator1 : Terminator
  Variable displacement motor 2 : variable_displacement_motor_2_lib/Variable displacement motor 2  max_Dv=Vm_nom cm^3/rev  min_Dv=20 cm^3/rev  inertia_motor=Jm kg*m^2  oil_vol=4.1 l  bulk=bulk Pa  bp=bm N*m*s/rad  lk=1e-6 m  t_specify=off  t_priority=None  t=0 N*m  t_nominal_specify=off  t_nominal_unit=N*m  t_nominal_value=1  q_specify=off  q_priority=None  q=0 m^3/s  q_nominal_specify=off  q_nominal_unit=m^3/s  q_nominal_value=1  qt_specify=off  qt_priority=None  qt=0 m^3/s  qt_nominal_specify=off  qt_nominal_unit=m^3/s  qt_nominal_value=1  qleak_specify=off  qleak_priority=None  qleak=0 m^3/s  qleak_nominal_specify=off  qleak_nominal_unit=m^3/s  qleak_nominal_value=1  Dv_specify=off  Dv_priority=None  Dv=0 cm^3/rev  Dv_nominal_specify=off  Dv_nominal_unit=cm^3/rev  Dv_nominal_value=1  dp_specify=off  dp_priority=None  dp=0 Pa  dp_nominal_specify=off  dp_nominal_unit=Pa  dp_nominal_value=1  wm_specify=off  wm_priority=None  wm=0 rad/s  wm_nominal_specify=off  wm_nominal_unit=rad/s  wm_nominal_value=1
      settings: InternalSimscapePortConfiguration="{\"Bottom\":[],\"Left\":[{\"id\":\"Vd\",\"label\":\"Vd\",\"type\":\"input\"},{\"id\":\"A\",\"label\":\"A\",\"type\":\"foundation.hydraulic.hydraulic\"},{\"id\":\"B\",\"label\":\"B\",\"type\":\"foundation.hydraulic.hydraulic\"}],\"Right\":[{\"id\":\"C\",\"label\":\"C\",\"type\":\"foundation.mechanical.rotational.rotational\"},{\"id\":\"q_out\",\"label\":\"q\",\"type\":\"output\"},{\"id\":\"delta_p_out\",\"label\":\"dp\",\"type\":\"output\"}],\"Top\":[]}"
  Variable displacement pump 2 : variable_displacement_pump_2_lib/Variable displacement pump 2  max_Dv=Vp_nom cm^3/rev  inertia_pump=Jp kg*m^2  oil_vol=3.0 l  bulk=bulk Pa  bp=bp N*m*s/rad  lk=1e-6 m  t_specify=off  t_priority=None  t=0 N*m  t_nominal_specify=off  t_nominal_unit=N*m  t_nominal_value=1  q_specify=off  q_priority=None  q=0 m^3/s  q_nominal_specify=off  q_nominal_unit=m^3/s  q_nominal_value=1  qt_specify=off  qt_priority=None  qt=0 m^3/s  qt_nominal_specify=off  qt_nominal_unit=m^3/s  qt_nominal_value=1  qleak_specify=off  qleak_priority=None  qleak=0 m^3/s  qleak_nominal_specify=off  qleak_nominal_unit=m^3/s  qleak_nominal_value=1  Dv_specify=off  Dv_priority=None  Dv=0 cm^3/rev  Dv_nominal_specify=off  Dv_nominal_unit=cm^3/rev  Dv_nominal_value=1  dp_specify=off  dp_priority=None  dp=0 Pa  dp_nominal_specify=off  dp_nominal_unit=Pa  dp_nominal_value=1  we_specify=off  we_priority=None  we=0 rad/s  we_nominal_specify=off  we_nominal_unit=rad/s  we_nominal_value=1
      settings: InternalSimscapePortConfiguration="{\"Bottom\":[],\"Left\":[{\"id\":\"Vd\",\"label\":\"Vd\",\"type\":\"input\"},{\"id\":\"C\",\"label\":\"C\",\"type\":\"foundation.mechanical.rotational.rotational\"}],\"Right\":[{\"id\":\"A\",\"label\":\"A\",\"type\":\"foundation.hydraulic.hydraulic\"},{\"id\":\"B\",\"label\":\"B\",\"type\":\"foundation.hydraulic.hydraulic\"}],\"Top\":[]}"
  charge_system : Subsystem
      settings: PortSchema="{\"entries\":[{\"content\":{\"sides\":[{\"content\":{\"connectorIds\":[]},\"type\":\"ConnectorPlacement.EquallySpacedRectSide\",\"uuid\":\"e48dc60c-7abd-410a-894b-273047c8aadd\"},{\"content\":{\"connectorIds\":[],\"side\":\"RIGHT\"},\"type\":\"ConnectorPlacement.EquallySpacedRectSide\",\"uuid\":\"1866d745-b28e-4187-be81-03bff766c239\"},{\"content\":{\"connectorIds\":[\"LConn1\"],\"side\":\"TOP\"},\"type\":\"ConnectorPlacement.EquallySpacedRectSide\",\"uuid\":\"a7856f22-1a7f-4c46-a37a-59c4b01a6b79\"},{\"content\":{\"connectorIds\":[\"RConn1\",\"RConn2\"],\"side\":\"BOTTOM\"},\"type\":\"ConnectorPlacement.EquallySpacedRectSide\",\"uuid\":\"6254cc6e-0892-4919-86d5-0180151530d1\"}]},\"type\":\"ConnectorPlacement.EquallySpacedConnector\",\"uuid\":\"a983534e-afc0-4bb2-9b1c-06b03353b26b\"}],\"packageUris\":[\"http://schema.mathworks.com/mf0/Connector/19700101\"],\"version\":\"1.0\"}"
  dp(bar) : nesl_utility/PS-Simulink Converter  PhysicalDomain=network_engine_domain  SubClassName=ps_output  LeftPortType=input  RightPortType=output  PseudoPeriodic=off  Frequencies=[]  Unit=bar  AffineConversion=on
      settings: SourceProductBaseCode=PW,SS
  q(l/min) : nesl_utility/PS-Simulink Converter  PhysicalDomain=network_engine_domain  SubClassName=ps_output  LeftPortType=input  RightPortType=output  PseudoPeriodic=off  Frequencies=[]  Unit=l/min  AffineConversion=on
      settings: SourceProductBaseCode=PW,SS
  vd_ctrl_motor : Subsystem
  vd_ctrl_pump : Subsystem
  s : PMIOPort  Side=Left
  q : PMIOPort  Port=2  Side=Right
  dp : PMIOPort  Port=3  Side=Right
  c : PMIOPort  Port=4  Side=Right
  hydroA : PMIOPort  Port=5  Side=Left
  hydroB : PMIOPort  Port=6  Side=Left
  wires:
  q(l/min)/1 -> Terminator1/1
  dp(bar)/1 -> Terminator/1
  [vd_p] -> vd_ctrl_pump/1(vd_ref)
  [vd_m] -> vd_ctrl_motor/1(vd_ref)
  connections:
  Hydraulic Flow Rate Sensor/RConn1 -- q(l/min)/LConn1
  Variable displacement pump 2/RConn1 -- hydroA/RConn1 -- charge_system/LConn1 -- Hydraulic Flow Rate Sensor/LConn1
  dp(bar)/LConn1 -- Hydraulic Pressure Sensor/RConn2
  Variable displacement motor 2/RConn3 -- dp/RConn1
  Variable displacement motor 2/RConn1 -- c/RConn1
  Variable displacement motor 2/RConn2 -- q/RConn1
  Variable displacement pump 2/LConn1 -- vd_ctrl_pump/RConn1
  Hydraulic Flow Rate Sensor/RConn2 -- Hydraulic Pressure Sensor/LConn1 -- Variable displacement motor 2/LConn2
  Variable displacement motor 2/LConn1 -- vd_ctrl_motor/RConn1
  s/RConn1 -- charge_system/RConn2 -- Variable displacement pump 2/LConn2
  Hydraulic Pressure Sensor/RConn1 -- Variable displacement motor 2/LConn3 -- charge_system/RConn1 -- hydroB/RConn1 -- Variable displacement pump 2/RConn2

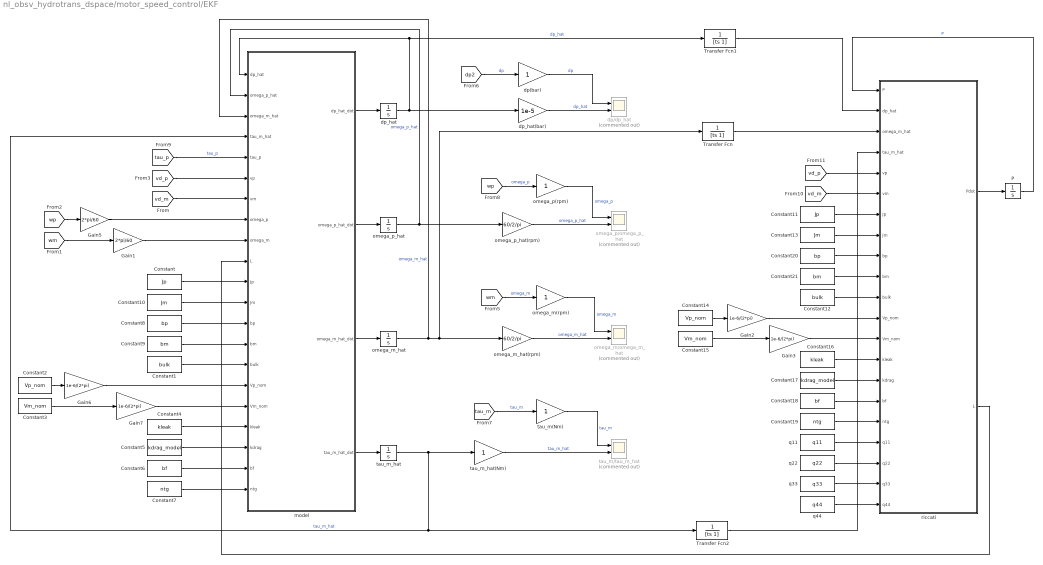
== system nl_obsv_hydrotrans_dspace/motor_speed_control/EKF ==
  Constant : Constant  Value=Jp
  Constant1 : Constant  Value=bulk
  Constant10 : Constant  Value=Jm
  Constant11 : Constant  Value=Jp
  Constant12 : Constant  Value=bulk
  Constant13 : Constant  Value=Jm
  Constant14 : Constant  Value=Vp_nom
  Constant15 : Constant  Value=Vm_nom
  Constant16 : Constant  Value=kleak
  Constant17 : Constant  Value=kdrag_model
  Constant18 : Constant  Value=bf
  Constant19 : Constant  Value=ntg
  Constant2 : Constant  Value=Vp_nom
  Constant20 : Constant  Value=bp
  Constant21 : Constant  Value=bm
  Constant3 : Constant  Value=Vm_nom
  Constant4 : Constant  Value=kleak
  Constant5 : Constant  Value=kdrag_model
  Constant6 : Constant  Value=bf
  Constant7 : Constant  Value=ntg
  Constant8 : Constant  Value=bp
  Constant9 : Constant  Value=bm
  Gain1 : Gain  Gain=2*pi/60
  Gain{2..3,6..7} (4 alike) : Gain  Gain=1e-6/(2*pi)
  Gain5 : Gain  Gain=2*pi/60
  P : Integrator  InitialCondition=P0
  Transfer Fcn : TransferFcn  Denominator=[ts 1]
  Transfer Fcn1 : TransferFcn  Denominator=[ts 1]
  Transfer Fcn2 : TransferFcn  Denominator=[ts 1]
  dp(bar) : Gain
  dp/dp_hat : Scope  Commented=on  NumInputPorts=2
  dp_hat : Integrator
  dp_hat(bar) : Gain  Gain=1e-5
  model : MATLAB Function  TreatAsAtomicUnit=on
  omega_m(rpm) : Gain
  omega_m/omega_m_hat : Scope  Commented=on  NumInputPorts=2
  omega_m_hat : Integrator
  omega_m_hat(rpm) : Gain  Gain=60/2/pi
  omega_p(rpm) : Gain
  omega_p/omega_p_hat : Scope  Commented=on  NumInputPorts=2
  omega_p_hat : Integrator
  omega_p_hat(rpm) : Gain  Gain=60/2/pi
  q11 : Constant  Value=q11
  q22 : Constant  Value=q22
  q33 : Constant  Value=q33
  q44 : Constant  Value=q44
  riccati : MATLAB Function  TreatAsAtomicUnit=on
  tau_m(Nm) : Gain
  tau_m/tau_m_hat : Scope  Commented=on  NumInputPorts=2
  tau_m_hat : Integrator
  tau_m_hat(Nm) : Gain
  wires:
  [wp] -> omega_p(rpm)/1  "omega_p"
  omega_p_hat(rpm)/1 -> omega_p/omega_p_hat/2  "omega_p_hat"
  [tau_m] -> tau_m(Nm)/1  "tau_m"
  omega_m_hat(rpm)/1 -> omega_m/omega_m_hat/2  "omega_m_hat"
  [wm] -> omega_m(rpm)/1  "omega_m"
  model/4(tau_m_hat_dot) -> tau_m_hat/1
  omega_m_hat/1 -> model/3(omega_m_hat), omega_m_hat(rpm)/1, Transfer Fcn/1  "omega_m_hat"
  model/3(omega_m_hat_dot) -> omega_m_hat/1
  [wm] -> Gain1/1
  [wp] -> Gain5/1
  model/1(dp_hat_dot) -> dp_hat/1
  dp_hat/1 -> dp_hat(bar)/1, model/1(dp_hat), Transfer Fcn1/1  "dp_hat"
  model/2(omega_p_hat_dot) -> omega_p_hat/1
  [dp2] -> dp(bar)/1  "dp"
  dp_hat(bar)/1 -> dp/dp_hat/2  "dp_hat"
  tau_m_hat/1 -> Transfer Fcn2/1, model/4(tau_m_hat), tau_m_hat(Nm)/1  "tau_m_hat"
  omega_p_hat/1 -> model/2(omega_p_hat), omega_p_hat(rpm)/1  "omega_p_hat"
  [tau_p] -> model/5(tau_p)  "tau_p"
  Gain5/1 -> model/8(omega_p)
  Gain1/1 -> model/9(omega_m)
  Constant/1 -> model/11(Jp)
  Constant10/1 -> model/12(Jm)
  Constant1/1 -> model/15(bulk)
  Constant2/1 -> Gain6/1
  Gain6/1 -> model/16(Vp_nom)
  Constant3/1 -> Gain7/1
  Gain7/1 -> model/17(Vm_nom)
  Constant4/1 -> model/18(kleak)
  Constant5/1 -> model/19(kdrag)
  Constant7/1 -> model/21(ntg)
  Constant6/1 -> model/20(bf)
  Constant9/1 -> model/14(bm)
  Constant8/1 -> model/13(bp)
  [vd_m] -> model/7(vm)
  [vd_p] -> model/6(vp)
  Constant14/1 -> Gain2/1
  Gain2/1 -> riccati/12(Vp_nom)
  Gain3/1 -> riccati/13(Vm_nom)
  Constant15/1 -> Gain3/1
  Constant16/1 -> riccati/14(kleak)
  Constant17/1 -> riccati/15(kdrag)
  Constant18/1 -> riccati/16(bf)
  Constant19/1 -> riccati/17(ntg)
  Constant11/1 -> riccati/7(Jp)
  Constant13/1 -> riccati/8(Jm)
  Constant20/1 -> riccati/9(bp)
  Constant21/1 -> riccati/10(bm)
  Constant12/1 -> riccati/11(bulk)
  [vd_p] -> riccati/5(vp)
  [vd_m] -> riccati/6(vm)
  riccati/1(Pdot) -> P/1
  P/1 -> riccati/1(P)  "P"
  riccati/2(L) -> model/10(L)
  q11/1 -> riccati/18(q11)
  q22/1 -> riccati/19(q22)
  q33/1 -> riccati/20(q33)
  q44/1 -> riccati/21(q44)
  tau_m_hat(Nm)/1 -> tau_m/tau_m_hat/2  "tau_m_hat"
  dp(bar)/1 -> dp/dp_hat/1  "dp"
  omega_p(rpm)/1 -> omega_p/omega_p_hat/1  "omega_p"
  omega_m(rpm)/1 -> omega_m/omega_m_hat/1  "omega_m"
  tau_m(Nm)/1 -> tau_m/tau_m_hat/1  "tau_m"
  Transfer Fcn/1 -> riccati/3(omega_m_hat)
  Transfer Fcn1/1 -> riccati/2(dp_hat)
  Transfer Fcn2/1 -> riccati/4(tau_m_hat)

== system nl_obsv_hydrotrans_dspace/motor_speed_control/pi-ctrl ==
  x : Inport
  xref : Inport  Port=2
  1/Ti : Gain  Gain=kp  SaturateOnIntegerOverflow=on  OutDataTypeStr=Inherit: Same as input  ParamDataTypeStr=Inherit: Same as input
  Saturation : Saturate  UpperLimit=sat_pos  LowerLimit=sat_neg
  Sum1 : Sum  Inputs=+++  SaturateOnIntegerOverflow=on
  Sum2 : Sum  Inputs=-+  SaturateOnIntegerOverflow=on
  Sum3 : Sum  Inputs=-+  SaturateOnIntegerOverflow=on
  Unit Delay1 : UnitDelay  SampleTime=ts  HasFrameUpgradeWarning=on
  Unit Delay2 : UnitDelay  SampleTime=ts  HasFrameUpgradeWarning=on
  Unit Delay4 : UnitDelay  SampleTime=ts  HasFrameUpgradeWarning=on
  kp : Gain  Gain=ki*ts  SaturateOnIntegerOverflow=on  OutDataTypeStr=Inherit: Same as input  ParamDataTypeStr=Inherit: Same as input
  u : Outport
  wires:
  Saturation/1 -> Sum3/2, u/1
  Unit Delay4/1 -> Sum1/3
  Sum1/1 -> Saturation/1
  x/1 -> Unit Delay1/1
  Sum3/1 -> Unit Delay4/1
  1/Ti/1 -> Sum3/1, Sum1/1
  Sum2/1 -> 1/Ti/1, kp/1
  kp/1 -> Sum1/2
  xref/1 -> Unit Delay2/1
  Unit Delay1/1 -> Sum2/1
  Unit Delay2/1 -> Sum2/2
